simulink model "outer_loop"  (R2024b)
settings: Solver=VariableStepAuto  StartTime=0.0  StopTime=40  FixedStep=0.01  RelTol=1e-3
values from neighbouring files (symbols this model uses):
  Dc = [1 f2 f1 0]    [automate_3rd_order.m]    (also in partC_manual_pole_placement.m; partE_controller.m; part_c_best_controller.m = [1 13.2 60.53 0]; part_c_controller.m = [1.0000 9.3000 30.6029 0])
  Nc = [g2 g1 g0]    [automate_3rd_order.m]    (also in partC_manual_pole_placement.m; partE_controller.m; part_c_best_controller.m = [0 -412.604327666152 -189.765069551777 -25.7063369397218]; part_c_controller.m = [-162.0139 -90.1688 -33.3170])
settings Model: Creator=zaras  LastModifiedBy=zaras

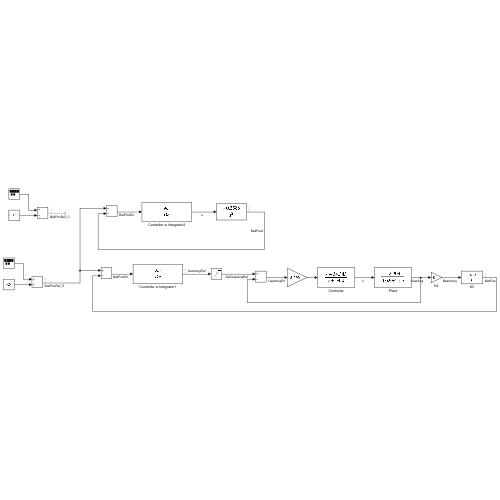
[thumbnail: Simulink's stored preview of the top-level diagram]
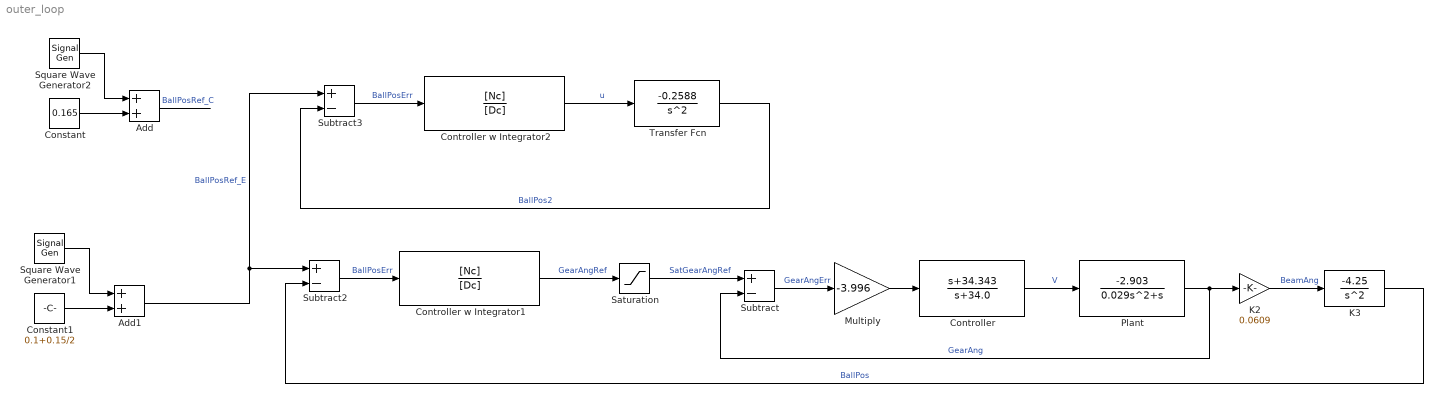
== system outer_loop ==
  Add : Sum
  Add1 : Sum
  Constant : Constant  Value=0.165
  Constant1 : Constant  Value=0.1+0.15/2
  Controller : TransferFcn  Numerator=[1 34.343]  Denominator=[1 34.0]
  Controller w Integrator1 : TransferFcn  Numerator=[Nc]  Denominator=[Dc]
  Controller w Integrator2 : TransferFcn  Numerator=[Nc]  Denominator=[Dc]
  K2 : Gain  Gain=0.0609
  K3 : TransferFcn  Numerator=[-4.25]  Denominator=[1 0 0]
  Multiply : Gain  Gain=-3.996
  Plant : TransferFcn  Numerator=[-2.903]  Denominator=[0.029 1 0]
  Saturation : Saturate  UpperLimit=0.785398  LowerLimit=-0.785398
  Square Wave Generator1 : SignalGenerator  WaveForm=square  Amplitude=0.15/2  Frequency=1/20
  Square Wave Generator2 : SignalGenerator  WaveForm=square  Amplitude=0.015  Frequency=1/20
  Subtract : Sum  Inputs=+-
  Subtract2 : Sum  Inputs=+-
  Subtract3 : Sum  Inputs=+-
  Transfer Fcn : TransferFcn  Numerator=[-0.2588]  Denominator=[1 0 0]
  wires:
  Square Wave Generator2/1 -> Add/1
  Constant/1 -> Add/2
  Controller w Integrator2/1 -> Transfer Fcn/1  "u"
  Subtract3/1 -> Controller w Integrator2/1  "BallPosErr"
  Transfer Fcn/1 -> Subtract3/2  "BallPos2"
  Saturation/1 -> Subtract/1  "SatGearAngRef"
  Multiply/1 -> Controller/1
  K2/1 -> K3/1  "BeamAng"
  Subtract2/1 -> Controller w Integrator1/1  "BallPosErr"
  Controller w Integrator1/1 -> Saturation/1  "GearAngRef"
  Subtract/1 -> Multiply/1  "GearAngErr"
  K3/1 -> Subtract2/2  "BallPos"
  Plant/1 -> Subtract/2, K2/1  "GearAng"
  Controller/1 -> Plant/1  "V"
  Add1/1 -> Subtract2/1, Subtract3/1  "BallPosRef_E"
  Constant1/1 -> Add1/2
  Square Wave Generator1/1 -> Add1/1
  Add/1 -> ?  "BallPosRef_C"
